simulink model "twolinkDynamics2012b"  (R2012b)
settings: Solver=ode45  SolverMode=SingleTasking  StartTime=0.0  StopTime=360  MaxStep=1  RelTol=1e-3
libraries: simulink x2
settings Model: SimulationMode=rapid-accelerator  CovMetricSettings=dwe  CovHtmlReporting=off  covSaveCumulativeToWorkspaceVar=off  CovSaveSingleToWorkspaceVar=off  CovExternalEMLEnable=on  Creator=ArsalanBangash  LastModifiedBy=ArsalanBangash
settings SolverCC: ZeroCrossControl=DisableAll
settings DataIOCC: LimitDataPoints=off  SaveFormat=StructureWithTime
settings OptimizationCC: ExpressionDepthLimit=128
settings DebuggingCC: UnderspecifiedInitializationDetection=Simplified  MergeDetectMultiDrivingBlocksExec=error  SolverPrmCheckMsg=none  FrameProcessingCompatibilityMsg=error  StateNameClashWarn=none  SFUnexpectedBacktrackingDiag=error  SFNoUnconditionalDefaultTransitionDiag=error
settings HardwareCC: ProdBitPerPointer=64  ProdLargestAtomicFloat=Float  ProdIntDivRoundTo=Zero  ProdEndianess=LittleEndian  ProdHWDeviceType=Specified
settings ModelReferenceCC: PropagateSignalLabelsOutOfModel=on
settings CodeAppCC: CustomSymbolStrType=$N$R$M_T
settings GRTTargetCC: CodeReplacementLibrary=C99 (ISO)  GeneratePreprocessorConditionals=Use local settings
settings ConfigurationSet: Description=SimMechanics 2G

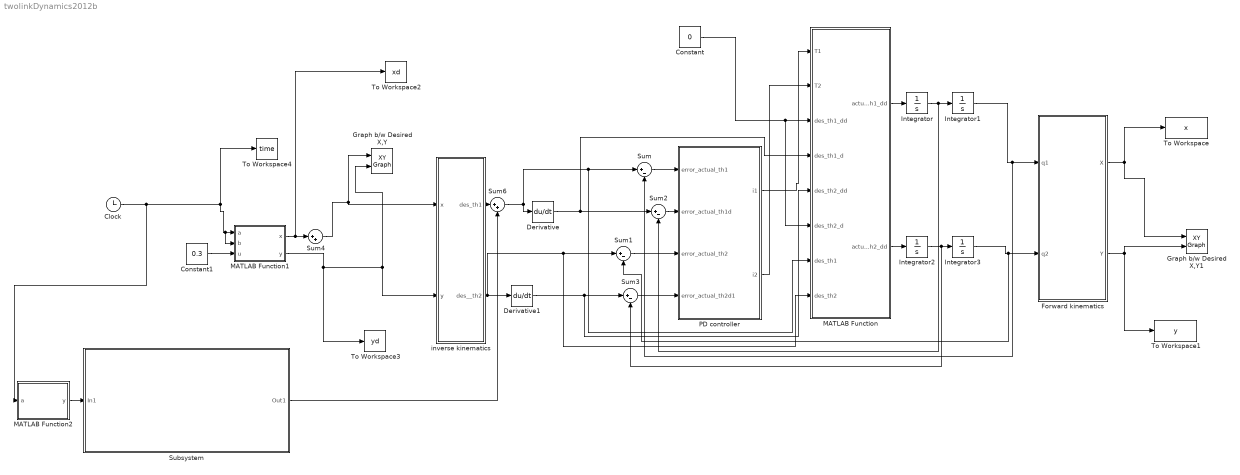
== system twolinkDynamics2012b ==
  Clock : Clock
  Constant : Constant  Value=0
  Constant1 : Constant  Value=0.3
  Derivative : Derivative
  Derivative1 : Derivative
  Forward kinematics : MATLAB Function  TreatAsAtomicUnit=on
  Graph b/w Desired X,Y : simulink/Sinks/XY Graph  xmin=0  xmax=2  ymin=0  ymax=2  st=1
  Graph b/w Desired X,Y1 : simulink/Sinks/XY Graph  xmin=0  xmax=2  ymin=0  ymax=2  st=1
  Integrator{,1..3} (4 alike) : Integrator
  MATLAB Function : MATLAB Function  TreatAsAtomicUnit=on
  MATLAB Function1 : MATLAB Function  TreatAsAtomicUnit=on
  MATLAB Function2 : MATLAB Function  TreatAsAtomicUnit=on
  PD controller : Subsystem
  Subsystem : Subsystem
  Sum{,1..3} (4 alike) : Sum  Inputs=|+-
  Sum4 : Sum  Inputs=|++
  Sum6 : Sum  Inputs=|++
  To Workspace : ToWorkspace  VariableName=x  SampleTime=-1
  To Workspace1 : ToWorkspace  VariableName=y  SampleTime=-1
  To Workspace2 : ToWorkspace  VariableName=xd  SampleTime=-1
  To Workspace3 : ToWorkspace  VariableName=yd  SampleTime=-1
  To Workspace4 : ToWorkspace  VariableName=time  SampleTime=-1
  inverse kinematics : MATLAB Function  TreatAsAtomicUnit=on
  wires:
  Sum6/1 -> MATLAB Function/7(des_th1), Sum/1, Derivative/1
  Sum/1 -> PD controller/1(error_actual_th1)
  Sum2/1 -> PD controller/2(error_actual_th1d)
  Sum1/1 -> PD controller/3(error_actual_th2)
  Sum3/1 -> PD controller/4(error_actual_th2d1)
  inverse kinematics/2(des__th2) -> Derivative1/1, MATLAB Function/8(des_th2), Sum1/1
  Derivative/1 -> MATLAB Function/4(des_th1_d), Sum2/1
  Derivative1/1 -> MATLAB Function/5(des_th2_dd), Sum3/1
  Sum4/1 -> inverse kinematics/1(x), Graph b/w Desired X,Y/1
  MATLAB Function1/2(y) -> To Workspace3/1, Graph b/w Desired X,Y/2, inverse kinematics/2(y)
  Forward kinematics/1(X) -> To Workspace/1, Graph b/w Desired X,Y1/1
  Forward kinematics/2(Y) -> Graph b/w Desired X,Y1/2, To Workspace1/1
  PD controller/2(i2) -> MATLAB Function/2(T2)
  Constant/1 -> MATLAB Function/6(des_th2_d), MATLAB Function/3(des_th1_dd)
  MATLAB Function/1(actual_th1_dd) -> Integrator/1
  Integrator/1 -> Sum2/2, Integrator1/1
  Integrator1/1 -> Sum/2, Forward kinematics/1(q1)
  MATLAB Function/2(actual_th2_dd) -> Integrator2/1
  Integrator2/1 -> Sum3/2, Integrator3/1
  Integrator3/1 -> Sum1/2, Forward kinematics/2(q2)
  Constant1/1 -> MATLAB Function1/3(u)
  Clock/1 -> MATLAB Function2/1(a), MATLAB Function1/2(b), MATLAB Function1/1(a), To Workspace4/1
  MATLAB Function1/1(x) -> To Workspace2/1, Sum4/1
  Subsystem/1(Out1) -> Sum6/2
  MATLAB Function2/1(y) -> Subsystem/1(In1)
  PD controller/1(i1) -> MATLAB Function/1(T1)
  inverse kinematics/1(des_th1) -> Sum6/1

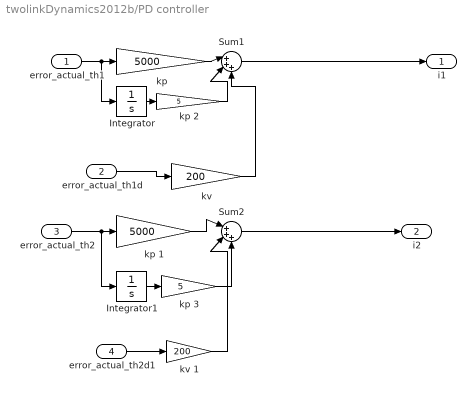
== system twolinkDynamics2012b/PD controller ==
  error_actual_th1 : Inport
  error_actual_th1d : Inport  Port=2
  error_actual_th2 : Inport  Port=3
  error_actual_th2d1 : Inport  Port=4
  Integrator : Integrator
  Integrator1 : Integrator
  Sum1 : Sum  Inputs=|+++
  Sum2 : Sum  Inputs=|+++
  "kp " : Gain  Gain=5000
  kp 1 : Gain  Gain=5000
  kp 2 : Gain  Gain=5
  kp 3 : Gain  Gain=5
  "kv " : Gain  Gain=200
  kv 1 : Gain  Gain=200
  i1 : Outport
  i2 : Outport  Port=2
  wires:
  Sum1/1 -> i1/1
  "kp "/1 -> Sum1/1
  error_actual_th1d/1 -> "kv "/1
  error_actual_th1/1 -> Integrator/1, "kp "/1
  "kv "/1 -> Sum1/3
  error_actual_th2/1 -> Integrator1/1, kp 1/1
  kv 1/1 -> Sum2/2
  error_actual_th2d1/1 -> kv 1/1
  kp 1/1 -> Sum2/1
  Sum2/1 -> i2/1
  Integrator/1 -> kp 2/1
  kp 2/1 -> Sum1/2
  Integrator1/1 -> kp 3/1
  kp 3/1 -> Sum2/3

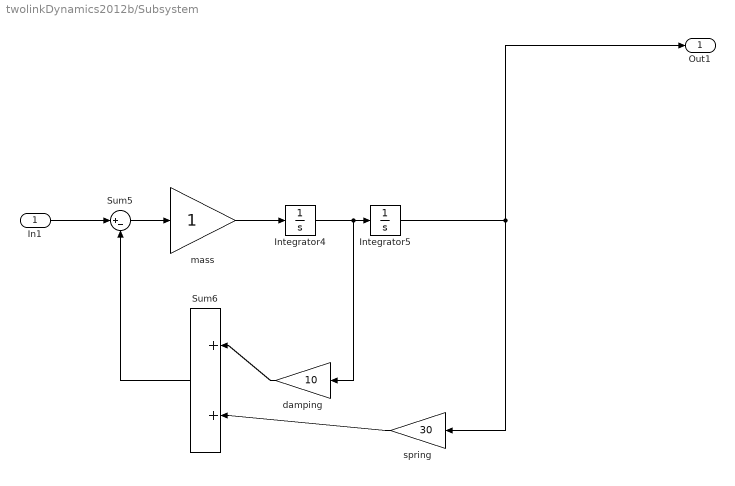
== system twolinkDynamics2012b/Subsystem ==
  In1 : Inport
  Integrator4 : Integrator
  Integrator5 : Integrator
  Sum5 : Sum  Inputs=|+-
  Sum6 : Sum  Inputs=|++
  damping : Gain  Gain=10
  mass : Gain
  spring : Gain  Gain=30
  Out1 : Outport
  wires:
  Sum5/1 -> mass/1
  mass/1 -> Integrator4/1
  Integrator4/1 -> damping/1, Integrator5/1
  spring/1 -> Sum6/2
  Integrator5/1 -> Out1/1, spring/1
  Sum6/1 -> Sum5/2
  damping/1 -> Sum6/1
  In1/1 -> Sum5/1

== matlab function twolinkDynamics2012b/Forward kinematics ==
  data: X output; Y output; q1 input; q2 input
function [X,Y]= fcn(q1,q2)
%#codegen
L1=2;
L2=2;
X=L2*cos(q1+q2) +L1*cos(q1);
Y=L2*sin(q1+q2) + L1*sin(q1);
end

== matlab function twolinkDynamics2012b/inverse kinematics ==
  data: x input; des_th1 output; y input; des__th2 output
function [des_th1,des__th2]= fcn(x,y)
L1=2;
L2=2;
M1=1;
M2=1;
c2= (x^2 +y^2 -L1^2 -L2^2)/(2*L1*L2)
s2=(1-c2^2)^0.5
K1= L1+L2*c2;
K2=L2*s2;
des_th1= atan2 (y,x)-atan2(K2,K1);
des__th2=atan2 (s2,c2);

== matlab function twolinkDynamics2012b/MATLAB Function ==
  data: T1 input; actual_th1_dd output; T2 input; des_th1_dd input; des_th1_d input; des_th2_dd input; des_th2_d input; des_th1 input; des_th2 input; actual_th2_dd output
function [actual_th1_dd,actual_th2_dd]= fcn(T1, T2,des_th1_dd,des_th1_d,des_th2_dd,des_th2_d,des_th1,des_th2)



N=1;
jm1=0.01;
jm2=0.01;
cm1=0.1;
cm2=0.1;
M1=1;
M2=0.5;
L1=2;
L2=1;
g=9.8;

th1=des_th1
th2=des_th2
th1dd=des_th1_dd
th1d=des_th1_d
th2dd=des_th2_dd
th2d=des_th2_d

M=[((M1+M2)*(L1^2)+ (M2*L2^2)+ (2*M2*L1*L2*cos(th2)))  (M2*L2^2+ M2*L1*L2*cos(th2));
   (M2*L2^2+M2*L1*L2*cos(th2))                   (M2*L2^2)];


V=[((-M2*L1*L2)*(2*th1d*th2d+th2d^2)*sin(th2));
   (M2*L1*L2*th1d^2*sin(th2))];




 G= [((M1+M2)*g*L1*cos(th1)+M2*g*L2*cos(th1+th2));
     M2*g*L2*cos(th1+th2)];
 
T=[T1;T2];
actual_th_dd= inv(M) *(T -V- G);
v= actual_th_dd(1)
w=actual_th_dd(2)

actual_th1_dd=v
actual_th2_dd=w

== matlab function twolinkDynamics2012b/MATLAB Function1 ==
  data: a input; b input; x output; u input; y output
function [x,y]= fcn(a,b,u)


x= 1 +u*cosd(a);
y=1+u*sind(b);

== matlab function twolinkDynamics2012b/MATLAB Function2 ==
  data: a input; y output
function y = fcn(a)
if a>=200 && a<=201
    y=1;
else
    y=0;
end
